simulink library "lib_TorqueDistribution_2017a"  (R2017a)
settings: Solver=VariableStepAuto  StartTime=0.0  StopTime=10.0  RelTol=1e-3
undefined symbols (not defined in the file): cal, eng, Engine, gb, mot
libraries: simulink x30, dspsigops x3, EC2_libraries x2
(part 1 of 4)
settings Model: Creator=Vraj M  LastModifiedBy=vraj

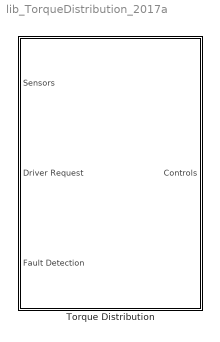
== system lib_TorqueDistribution_2017a ==
  Torque Distribution : Subsystem

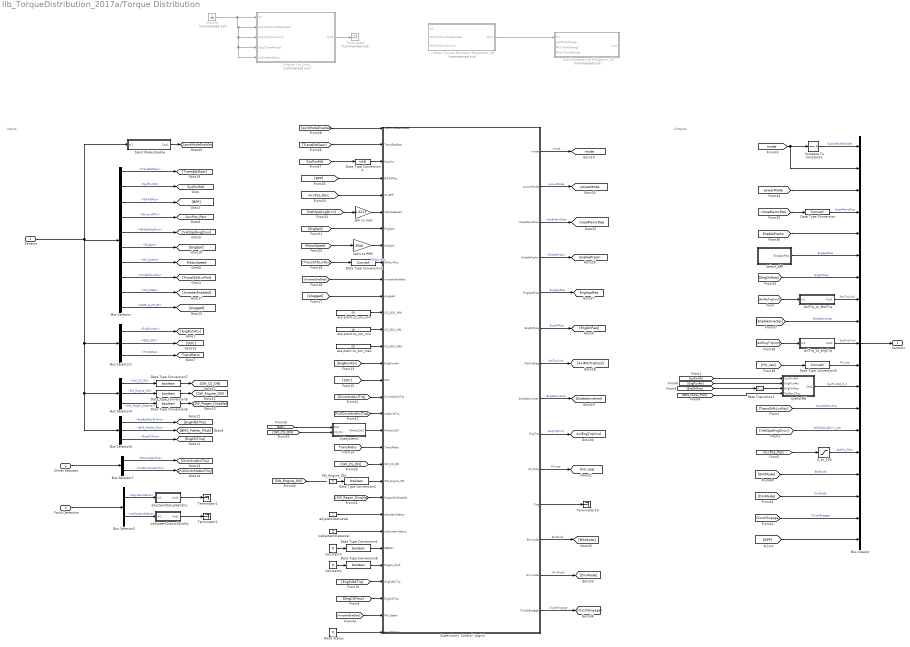
== system lib_TorqueDistribution_2017a/Torque Distribution ==
  note: Inputs
  note: Outputs
  Sensors : Inport
  Driver Request : Inport  Port=2
  Fault Detection : Inport  Port=3
  0_to_100 : Saturate  UpperLimit=100  LowerLimit=0
  AxlTrq_to_EngTrq : Subsystem
  AxlTrq_to_MotTrq : Subsystem
  Bus Creator : BusCreator  Inputs=19
  Bus Selector : BusSelector  OutputSignals=from_CAN.fromVEH_CAN.from_TCM.TransEstGear,from_CAN.fromVEH_CAN.from_BCM.SysPwrMd,from_CAN.fromVEH_CAN.from_BCM.BrkPdlPos,from_Analog.Driver_APP1,from_CAN.fromEBCAN.from_ECM.VehSpdAvgDrvn,from_CAN.fromEBCAN.from_ECM.EngSpd,from_CAN.fromHV_CAN.from_MCU.INV_VCU_01.INV_Speed,from_CAN.fromVEH_CAN.from_TCM.TrnsShftLvrPos,from_CAN.fromHV_CAN.from_MCU.INV_VCU_01.INV_State,from_CAN.fromHV_CAN.from_OBC.NLG5_ST.NLG5_S_CP_DT
  Bus Selector1 : BusSelector  OutputSignals=from_CAN.fromEBCAN.from_ECM.EngRunAtv,from_CAN.fromHV_CAN.from_BMSHybrid.BMS_SOC,from_CAN.fromVEH_CAN.from_TCM.TrnGrRat
  Bus Selector2 : BusSelector  OutputSignals=eSystemDiagOut.eSystemStatus,iceSystemDiagOut.iceSystemStatus
  Bus Selector4 : BusSelector  OutputSignals=from_Digital.SW_CS_ON,from_Digital.SW_Engine_ON,from_Digital.SW_Regen_Disable
  Bus Selector6 : BusSelector  OutputSignals=from_CAN.fromEBCAN.from_ECM.EngActStdyStTorq,from_CAN.fromHV_CAN.from_BMSHybrid.BMS_HYB_02.BMS_Fehler_Pilot,from_CAN.fromEBCAN.from_ECM.EngCltTmp
  Bus Selector7 : BusSelector  OutputSignals=DrvIntndAxlTrq,FullDrvIntndAxlTrq
  Compare To Constant1 : simulink/Logic and Bit Operations/Compare To Constant  relop===  const=4  OutDataTypeStr=boolean
  Constant2 : Constant  Value=0
  Constant3 : Constant  Value=0
  Data Type Conversion : DataTypeConversion
  Data Type Conversion{1..2,5..8} (6 alike) : DataTypeConversion  OutDataTypeStr=boolean
  Data Type Conversion3 : DataTypeConversion
  Data Type Conversion4 : DataTypeConversion  OutDataTypeStr=int8
  Data Type Conversion9 : DataTypeConversion
  Engine Trq Limit : Subsystem  Commented=on
  Ground : Ground  Commented=on
  Hood Status : Constant  Value=0
  Motor Troque Mismatch Mitigation_CD : Subsystem  Commented=on
  OverTemperature Mitigation_CD : Subsystem  Commented=on
  Rate Transition3 : RateTransition
  SW_Engine_ON : Constant  Value=0
  Select_APP : Subsystem
  Sport Mode Enable : Subsystem
  Subsystem1 : Subsystem
  Supervisory  Control  Logic1 : Stateflow chart  TreatAsAtomicUnit=on
  SysPwrMd : Subsystem
  Terminator : Terminator  Commented=on
  Terminator1 : Terminator
  Terminator10 : Terminator
  Terminator2 : Terminator
  eSystemStatusVal : Constant  Value=2
  eSystemStatusValidity : Subsystem
  ess.plant.cd_soc_min : Constant  Value=50
  ess.plant.cs_soc_max : Constant  Value=23
  ess.plant.cs_soc_min : Constant  Value=18
  iceSystemStatusVal : Constant  Value=2
  iceSystemStatusValidity : Subsystem
  kph to mph : Gain  Gain=0.6213
  rad/s to RPM : Gain  Gain=30/pi
  Controls : Outport
  tag scope: AccPos_Perc=global, AxlEngTrqCmd=global, EnablePrplsn=global, EngAppReq=global, MotorSpeed=global, SportModeEnabled=global, SysPwrMd=global, TransRatio=global, closeMaincReq=global, mode=global, powerMode=global
  wires:
  Hood Status/1 -> Supervisory  Control  Logic1/31(HoodStatus)
  Ground/1 -> Engine Trq Limit/1(In1), Engine Trq Limit/2(EngTrqMismchDegraded), Engine Trq Limit/3(EngTrqMismchLimp), Engine Trq Limit/4(Eng_TempRange), Engine Trq Limit/5(iceSystemStatus)
  [plugged] -> Supervisory  Control  Logic1/11(plugged)
  AxlTrq_to_EngTrq/1(Out1) -> Bus Creator/10  "EngTrqCmd"
  [closeMaincReq] -> Data Type Conversion/1
  Compare To Constant1/1 -> Bus Creator/1  "SportsModeEnable"
  [EngRunAtv] -> SysPwrMd/2(EngRunAtv)
  [ClutchEngage] -> Bus Creator/18  "ClutchEngage"
  [BPP] -> Bus Creator/19
  [AxlMtrTrqCmd] -> AxlTrq_to_MotTrq/1(In1)
  [AxlEngTrqCmd] -> AxlTrq_to_EngTrq/1(In1)
  [mode] -> Compare To Constant1/1, Bus Creator/2
  [TransShftLvrPos] -> Bus Creator/13  "TransShftLvrPos"
  [DrvMode] -> Bus Creator/17  "DrvMode"
  [SysPwrMd] -> SysPwrMd/1(SysPwrMd)
  SysPwrMd/1(Out1) -> Bus Creator/12  "SysPwrMd_0_3"
  [VehSpdAvgDrvn] -> Bus Creator/14  "VehSpdAvgDrvn_kph"
  Data Type Conversion9/1 -> Bus Creator/11  "HV_req"
  [BMS_Fehler_Pilot] -> SysPwrMd/4(Fehler_Pilot)
  [EnablePrplsn] -> Bus Creator/5
  [AccPos_Perc] -> 0_to_100/1
  [EnableInverter] -> Bus Creator/9  "EnableInverter"
  [EngOnReq] -> Bus Creator/7  "EngOnReq"
  [HV_req] -> Data Type Conversion9/1
  Select_APP/1(EngAppReq) -> Bus Creator/6  "EngAppReq"
  [BrkMode] -> Bus Creator/16  "BrkMode"
  AxlTrq_to_MotTrq/1(Out1) -> Bus Creator/8  "MtrTrqCmd"
  0_to_100/1 -> Bus Creator/15  "AccPos_Perc"
  [powerMode] -> Bus Creator/3
  Data Type Conversion/1 -> Bus Creator/4  "closeMaincReq"
  [EngOnReq] -> Rate Transition3/1
  Rate Transition3/1 -> SysPwrMd/3(EngOnReq)
  Bus Creator/1 -> Controls/1
  Sensors/1 -> Bus Selector/1, Sport Mode Enable/1(In1), Bus Selector1/1, Bus Selector4/1, Bus Selector6/1
  Bus Selector/1 -> [TransEstGear]  "<TransEstGear>"
  Bus Selector/2 -> [SysPwrMd]  "<SysPwrMd>"
  Bus Selector/3 -> [BPP]  "<BrkPdlPos>"
  Bus Selector/4 -> [AccPos_Perc]  "<Driver_APP1>"
  Bus Selector/5 -> [VehSpdAvgDrvn]  "<VehSpdAvgDrvn>"
  Bus Selector/6 -> [EngSpd]  "<EngSpd>"
  Bus Selector/7 -> [MotorSpeed]  "<INV_Speed>"
  Bus Selector/9 -> [InverterEnabled]  "<INV_State>"
  Bus Selector1/1 -> [EngRunAtv]  "<EngRunAtv>"
  Bus Selector/8 -> [TransShftLvrPos]  "<TrnsShftLvrPos>"
  Bus Selector1/3 -> [TransRatio]  "<TrnGrRat>"
  Fault Detection/1 -> Bus Selector2/1
  Bus Selector2/1 -> eSystemStatusValidity/1(In1)  "<eSystemStatus>"
  Bus Selector2/2 -> iceSystemStatusValidity/1(In1)  "<iceSystemStatus>"
  Bus Selector4/3 -> Data Type Conversion6/1  "<SW_Regen_Disable>"
  Bus Selector4/1 -> Data Type Conversion7/1  "<SW_CS_ON>"
  Bus Selector4/2 -> Data Type Conversion5/1  "<SW_Engine_ON>"
  eSystemStatusValidity/1(Out1) -> Terminator1/1
  iceSystemStatusValidity/1(Out1) -> Terminator2/1
  Bus Selector/10 -> [plugged]  "<NLG5_S_CP_DT>"
  Data Type Conversion5/1 -> [SW_Engine_ON]
  Data Type Conversion6/1 -> [SW_Regen_Disable]
  Bus Selector6/1 -> [EngFdbkTrq]  "<EngActStdyStTorq>"
  Bus Selector6/2 -> [BMS_Fehler_Pilot]  "<BMS_Fehler_Pilot>"
  Bus Selector6/3 -> [EngCltTmp]  "<EngCltTmp>"
  Bus Selector7/2 -> [FullDrvIntndAxlTrq]  "<FullDrvIntndAxlTrq>"
  Sport Mode Enable/1(Out1) -> [SportModeEnabled]
  Bus Selector1/2 -> [SOC]  "<BMS_SOC>"
  Data Type Conversion7/1 -> [SW_CS_ON]
  Driver Request/1 -> Bus Selector7/1
  Bus Selector7/1 -> [DrvIntndAxlTrq]  "<DrvIntndAxlTrq>"
  Supervisory  Control  Logic1/14(ClutchEngage) -> [ClutchEngage]  "ClutchEngage"
  Supervisory  Control  Logic1/13(Drvmode) -> [DrvMode]  "DrvMode"
  Supervisory  Control  Logic1/10(HV_Req) -> [HV_req]  "HV_req"
  Supervisory  Control  Logic1/9(EngTrq) -> [AxlEngTrqCmd]  "EngTrqCmd"
  Supervisory  Control  Logic1/7(MotTrqReq) -> [AxlMtrTrqCmd]  "MtrTrqCmd"
  Supervisory  Control  Logic1/6(EngOnReq) -> [EngOnReq]  "EngOnReq"
  [SW_CS_ON] -> Subsystem1/2(CS_On)
  [SW_Regen_Disable] -> Supervisory  Control  Logic1/23(RegenBrkDisable)
  [SW_Engine_ON] -> ?
  [SW_CS_ON] -> Supervisory  Control  Logic1/21(SW_CS_ON)
  [SportModeEnabled] -> Supervisory  Control  Logic1/1(SportModeEnabled)
  Data Type Conversion4/1 -> Supervisory  Control  Logic1/3(KeyPos)
  [SysPwrMd] -> Data Type Conversion4/1
  [TransEstGear] -> Supervisory  Control  Logic1/2(TransEstGear)
  [BPP] -> Supervisory  Control  Logic1/4(BrkPdlPos)
  [AccPos_Perc] -> Supervisory  Control  Logic1/5(drvAPP)
  [VehSpdAvgDrvn] -> kph to mph/1
  [EngSpd] -> Supervisory  Control  Logic1/7(EngSpd)
  [MotorSpeed] -> rad/s to RPM/1
  [TransShftLvrPos] -> Data Type Conversion3/1
  [InverterEnabled] -> Supervisory  Control  Logic1/10(InverterEnabled)
  [SOC] -> Subsystem1/1(SoC)
  [SOC] -> Supervisory  Control  Logic1/16(SoC)
  [TransRatio] -> Supervisory  Control  Logic1/20(TransRatio)
  [EngRunAtv] -> Supervisory  Control  Logic1/15(EngRunAtv)
  [EngFdbkTrq] -> Supervisory  Control  Logic1/28(EngFdbkTrq)
  [EngCltTmp] -> Supervisory  Control  Logic1/29(EngCtlTmp)
  rad/s to RPM/1 -> Supervisory  Control  Logic1/8(MotSpd)
  Supervisory  Control  Logic1/5(EngAppReq) -> [EngAppReq]  "EngAppReq"
  eSystemStatusVal/1 -> Supervisory  Control  Logic1/24(eSystemStatus)
  iceSystemStatusVal/1 -> Supervisory  Control  Logic1/25(iceSystemStatus)
  Data Type Conversion8/1 -> Supervisory  Control  Logic1/27(Regen_fault)
  Supervisory  Control  Logic1/12(Brkmode) -> [BrkMode]  "BrkMode"
  Subsystem1/1(Faked_SoC) -> Supervisory  Control  Logic1/19(Faked_SoC)
  Data Type Conversion1/1 -> Supervisory  Control  Logic1/26(ABSAtv)
  Constant3/1 -> Data Type Conversion1/1
  [FullDrvIntndAxlTrq] -> Supervisory  Control  Logic1/18(IntdAxleTrq)
  [DrvIntndAxlTrq] -> Supervisory  Control  Logic1/17(DrvIntdAxleTrq)
  Supervisory  Control  Logic1/11(Chg) -> Terminator10/1
  Motor Troque Mismatch Mitigation_CD/1(Out1) -> OverTemperature Mitigation_CD/1(In1)
  Engine Trq Limit/1(Out1) -> Terminator/1
  Constant2/1 -> Data Type Conversion8/1
  kph to mph/1 -> Supervisory  Control  Logic1/6(VehicleSpeed)
  Data Type Conversion3/1 -> Supervisory  Control  Logic1/9(ShftLvrPos)  "ShftLvrPos"
  Supervisory  Control  Logic1/1(mode) -> [mode]  "mode"
  Supervisory  Control  Logic1/2(powerMode) -> [powerMode]  "powerMode"
  Supervisory  Control  Logic1/3(closeMaincReq) -> [closeMaincReq]  "closeMaincReq"
  Supervisory  Control  Logic1/4(EnablePrplsn) -> [EnablePrplsn]  "EnablePrplsn"
  Supervisory  Control  Logic1/8(EnableInverter) -> [EnableInverter]  "EnableInverter"
  ess.plant.cs_soc_max/1 -> Supervisory  Control  Logic1/14(CS_SOC_MAX)
  ess.plant.cs_soc_min/1 -> Supervisory  Control  Logic1/13(CS_SOC_MIN)
  ess.plant.cd_soc_min/1 -> Supervisory  Control  Logic1/12(CD_SOC_MIN)
  SW_Engine_ON/1 -> Data Type Conversion2/1
  Data Type Conversion2/1 -> Supervisory  Control  Logic1/22(SW_Engine_ON)
  [InverterEnabled] -> Supervisory  Control  Logic1/30(INV_State)

== system lib_TorqueDistribution_2017a/Torque Distribution/AxlTrq_to_EngTrq ==
  note: //From engine axle torque to engine torque//
  note: check this rate limiter
  In1 : Inport
  Compare To Constant : simulink/Logic and Bit Operations/Compare To Constant  relop===  const=0  OutDataTypeStr=boolean
  Constant1 : Constant  Value=max(gb.plant.init.ratio.map)
  Constant5 : Constant  Value=fd.plant.init.ratio
  Divide1 : Product  Inputs=*//
  Ground : Ground  Commented=on
  Rate Limiter : RateLimiter  RisingSlewLimit=1000  FallingSlewLimit=-2000
  Rate Limiter1 : RateLimiter  Commented=on  RisingSlewLimit=Engine.trq_uprate  FallingSlewLimit=Engine.trq_derate
  Ratio Filter : Subsystem
  Switch : Switch  Criteria=u2 > Threshold
  Terminator : Terminator  Commented=on
  Out1 : Outport
  wires:
  Ground/1 -> Rate Limiter1/1
  Rate Limiter1/1 -> Terminator/1
  Ratio Filter/1(Filtered_Ratio) -> Compare To Constant/1, Switch/3
  Rate Limiter/1 -> Out1/1
  Switch/1 -> Divide1/3
  Constant1/1 -> Switch/1
  Compare To Constant/1 -> Switch/2
  [TransRatio] -> Ratio Filter/1(Ratio)
  Divide1/1 -> Rate Limiter/1
  Constant5/1 -> Divide1/2
  In1/1 -> Divide1/1

== system lib_TorqueDistribution_2017a/Torque Distribution/AxlTrq_to_MotTrq ==
  In1 : Inport
  AxlTrq_to_MtrTrq2 : Subsystem
  MotTrqLimit : Saturate  UpperLimit=250  LowerLimit=-200
  Scope : Scope  NumInputPorts=4
  Subsystem : Subsystem
  electric machine filter : Subsystem
  Out1 : Outport
  wires:
  [MotorSpeed] -> Subsystem/2(RPM)
  MotTrqLimit/1 -> Subsystem/1(In1), Scope/3  "MtrTrqCmd"
  Subsystem/1(Out1) -> Out1/1, Scope/4  "MtrTrqCmd"
  electric machine filter/1(filtered) -> MotTrqLimit/1, Scope/2  "MtrTrqCmd"
  AxlTrq_to_MtrTrq2/1(MtrTrqCmd) -> electric machine filter/1(trq), Scope/1  "MtrTrqCmd"
  In1/1 -> AxlTrq_to_MtrTrq2/1(In1)

== system lib_TorqueDistribution_2017a/Torque Distribution/Engine Trq Limit ==
  In1 : Inport
  EngTrqMismchDegraded : Inport  Port=2
  EngTrqMismchLimp : Inport  Port=3
  Eng_TempRange : Inport  Port=4
  iceSystemStatus : Inport  Port=5
  Compare To Constant : simulink/Logic and Bit Operations/Compare To Constant  relop===  const=1  OutDataTypeStr=boolean
  Eng Troque Mismatch Mitigation : Subsystem
  OverTemperature Mitigation : Subsystem
  Switch2 : Switch  Threshold=1
  Out1 : Outport
  wires:
  OverTemperature Mitigation/1(Out1) -> Switch2/1
  iceSystemStatus/1 -> Compare To Constant/1
  In1/1 -> Switch2/3, Eng Troque Mismatch Mitigation/1(In1)
  Eng Troque Mismatch Mitigation/1(Out1) -> OverTemperature Mitigation/1(In1)
  Eng_TempRange/1 -> OverTemperature Mitigation/2(essTempRange)
  EngTrqMismchDegraded/1 -> Eng Troque Mismatch Mitigation/2(EngTrqMismchDegraded)
  EngTrqMismchLimp/1 -> Eng Troque Mismatch Mitigation/3(EngTrqMismchLimp)
  Compare To Constant/1 -> Switch2/2
  Switch2/1 -> Out1/1

== system lib_TorqueDistribution_2017a/Torque Distribution/Motor Troque Mismatch Mitigation_CD ==
  In1 : Inport
  MotTrqMismchDegraded : Inport  Port=2
  MotTrqMismchLimp : Inport  Port=3
  Subsystem : Subsystem
  Out1 : Outport
  tag scope: TorqueRequest_Nm=global
  wires:
  Subsystem/1(Out1) -> Out1/1
  MotTrqMismchDegraded/1 -> Subsystem/2(In2)
  MotTrqMismchLimp/1 -> Subsystem/1(In1)
  In1/1 -> [TorqueRequest_Nm]

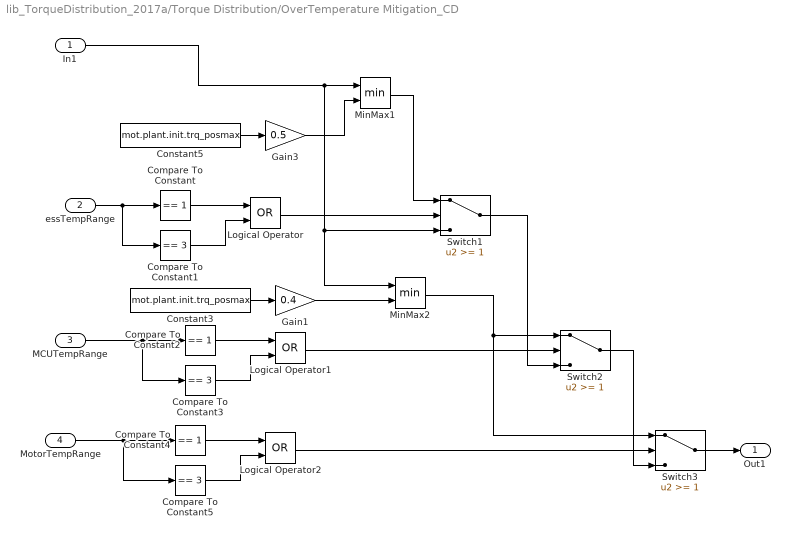
== system lib_TorqueDistribution_2017a/Torque Distribution/OverTemperature Mitigation_CD ==
  In1 : Inport
  essTempRange : Inport  Port=2
  MCUTempRange : Inport  Port=3
  MotorTempRange : Inport  Port=4
  Compare To Constant : simulink/Logic and Bit Operations/Compare To Constant  relop===  const=1  OutDataTypeStr=boolean
  Compare To Constant1 : simulink/Logic and Bit Operations/Compare To Constant  relop===  const=3  OutDataTypeStr=boolean
  Compare To Constant2 : simulink/Logic and Bit Operations/Compare To Constant  relop===  const=1  OutDataTypeStr=boolean
  Compare To Constant3 : simulink/Logic and Bit Operations/Compare To Constant  relop===  const=3  OutDataTypeStr=boolean
  Compare To Constant4 : simulink/Logic and Bit Operations/Compare To Constant  relop===  const=1  OutDataTypeStr=boolean
  Compare To Constant5 : simulink/Logic and Bit Operations/Compare To Constant  relop===  const=3  OutDataTypeStr=boolean
  Constant3 : Constant  Value=mot.plant.init.trq_posmax
  Constant5 : Constant  Value=mot.plant.init.trq_posmax
  Gain1 : Gain  Gain=0.4
  Gain3 : Gain  Gain=0.5
  Logical Operator : Logic  Operator=OR  AllPortsSameDT=off  OutDataTypeStr=boolean
  Logical Operator1 : Logic  Operator=OR  AllPortsSameDT=off  OutDataTypeStr=boolean
  Logical Operator2 : Logic  Operator=OR  AllPortsSameDT=off  OutDataTypeStr=boolean
  MinMax1 : MinMax  Inputs=2
  MinMax2 : MinMax  Inputs=2
  Switch1 : Switch  Threshold=1
  Switch2 : Switch  Threshold=1
  Switch3 : Switch  Threshold=1
  Out1 : Outport
  wires:
  Switch3/1 -> Out1/1
  Compare To Constant5/1 -> Logical Operator2/2
  Compare To Constant4/1 -> Logical Operator2/1
  Switch1/1 -> Switch2/3
  essTempRange/1 -> Compare To Constant/1, Compare To Constant1/1
  Compare To Constant3/1 -> Logical Operator1/2
  Compare To Constant2/1 -> Logical Operator1/1
  MCUTempRange/1 -> Compare To Constant2/1, Compare To Constant3/1
  Switch2/1 -> Switch3/3
  Gain3/1 -> MinMax1/2
  Gain1/1 -> MinMax2/2
  In1/1 -> MinMax1/1, Switch1/3, MinMax2/1
  Logical Operator2/1 -> Switch3/2
  Logical Operator/1 -> Switch1/2
  MinMax1/1 -> Switch1/1
  MinMax2/1 -> Switch2/1, Switch3/1
  Constant3/1 -> Gain1/1
  Compare To Constant/1 -> Logical Operator/1
  Compare To Constant1/1 -> Logical Operator/2
  Logical Operator1/1 -> Switch2/2
  Constant5/1 -> Gain3/1
  MotorTempRange/1 -> Compare To Constant4/1, Compare To Constant5/1

== system lib_TorqueDistribution_2017a/Torque Distribution/Select_APP ==
  APP_Select : Constant  Value=0
  Data Type Conversion10 : DataTypeConversion  OutDataTypeStr=boolean
  Switch1 : Switch  Criteria=u2 > Threshold
  EngAppReq : Outport
  wires:
  [EngAppReq] -> Switch1/3
  [AccPos_Perc] -> Switch1/1
  Data Type Conversion10/1 -> Switch1/2
  APP_Select/1 -> Data Type Conversion10/1
  Switch1/1 -> EngAppReq/1  "EngAppReq"

== system lib_TorqueDistribution_2017a/Torque Distribution/Sport Mode Enable ==
  In1 : Inport
  Bus Selector5 : BusSelector  OutputSignals=from_Analog.Sport_Mode_SW
  Compare To Constant : simulink/Logic and Bit Operations/Compare To Constant  relop===  const=2  OutDataTypeStr=boolean
  Sports Mode Logic : Stateflow chart  TreatAsAtomicUnit=on
  Out1 : Outport
  wires:
  In1/1 -> Bus Selector5/1
  Bus Selector5/1 -> Sports Mode Logic/1(Voltage_Input)  "<Sport_Mode_SW>"
  Sports Mode Logic/1(Driver_Mode) -> Compare To Constant/1
  Compare To Constant/1 -> Out1/1

== system lib_TorqueDistribution_2017a/Torque Distribution/Subsystem1 ==
  SoC : Inport
  CS_On : Inport  Port=2
  Constant : Constant
  Sample and Hold1 : dspsigops/Sample and Hold  trig=Rising edge  initCond=0  latchinput=off
  Switch : Switch  Criteria=u2 > Threshold
  Faked_SoC : Outport
  wires:
  SoC/1 -> Sample and Hold1/1
  CS_On/1 -> Switch/2, Sample and Hold1/Trigger
  Switch/1 -> Faked_SoC/1
  Sample and Hold1/1 -> Switch/1
  Constant/1 -> Switch/3

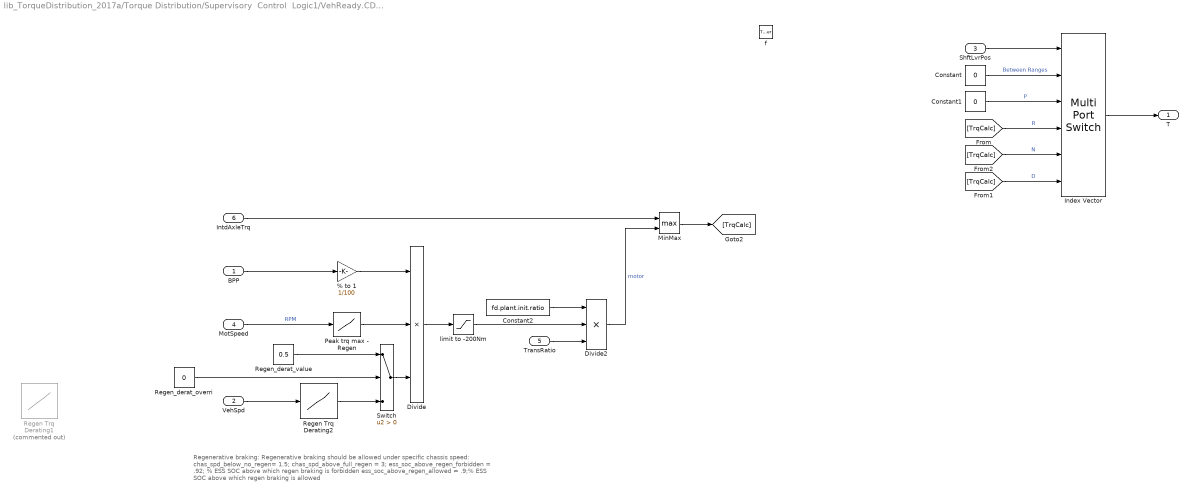
== system lib_TorqueDistribution_2017a/Torque Distribution/Supervisory  Control  Logic1/VehReady.CD_Mode.Brake_mode.MotTrqCalc1 ==
  note: Regenerative braking:
      | Regenerative braking should be allowed under specific chassis speed:
      | chas_spd_below_no_regen= 1.5;
      | chas_spd_above_full_regen = 3;
      | ess_soc_above_regen_forbidden = .92;  % ESS SOC above which regen braking is forbidden
      | ess_soc_above_regen_allowed = .9;% ESS SOC above which regen braking is allowed
  BPP : Inport
  VehSpd : Inport  Port=2
  ShftLvrPos : Inport  Port=3
  MotSpeed : Inport  Port=4
  TransRatio : Inport  Port=5
  IntdAxleTrq : Inport  Port=6
  f : TriggerPort  TriggerType=function-call  VariantControl=Variant
      settings: CopyFcn=Stateflow.SLINSF.SimulinkMan.removeBlockPreDeleteFcn  PreDeleteFcn=Stateflow.SLINSF.SimulinkMan.unsafePredeleteFcn
  "% to 1 " : Gain  Gain=1/100
  Constant : Constant  Value=0
  Constant1 : Constant  Value=0
  Constant2 : Constant  Value=fd.plant.init.ratio
  Divide : Product  Inputs=***
  Divide2 : Product  Inputs=***
  Index Vector : MultiPortSwitch  DataPortOrder=Zero-based contiguous  Inputs=5  zeroidx=on
  MinMax : MinMax  Function=max  Inputs=2
  Peak trq max - Regen : Lookup  InputValues=mot.plant.init.regen.trq_max.idx1_spd  Table=mot.plant.init.regen.trq_max.map  LookUpMeth=Interpolation-Use End Values  SaturateOnIntegerOverflow=on
  Regen Trq Derating1 : Lookup_n-D  Commented=on  NumberOfTableDimensions=1  BreakpointsForDimension1=[0 10 20 30 40]  Table=[0 0.025 0.05 0.1 1]  ExtrapMethod=Clip  UseLastTableValue=on  InternalRulePriority=Speed  RndMeth=Simplest  InputSameDT=on
  Regen Trq Derating2 : Lookup_n-D  NumberOfTableDimensions=1  BreakpointsForDimension1=[0 10 11 200]  Table=[0 0.5 1 1]  ExtrapMethod=Clip  UseLastTableValue=on  InternalRulePriority=Speed  RndMeth=Simplest  InputSameDT=on
  Regen_derat_overri : Constant  Value=0
  Regen_derat_value : Constant  Value=0.5
  Switch : Switch  Criteria=u2 > Threshold
  limit to -200Nm : Saturate  UpperLimit=0  LowerLimit=-200
  T : Outport
  wires:
  MinMax/1 -> [TrqCalc]
  IntdAxleTrq/1 -> MinMax/1
  Regen_derat_value/1 -> Switch/1
  Switch/1 -> Divide/3
  Regen_derat_overri/1 -> Switch/2
  Regen Trq Derating2/1 -> Switch/3
  Divide2/1 -> MinMax/2  "motor"
  TransRatio/1 -> Divide2/3
  limit to -200Nm/1 -> Divide2/2
  Constant2/1 -> Divide2/1
  Peak trq max - Regen/1 -> Divide/2
  MotSpeed/1 -> Peak trq max - Regen/1  "RPM"
  [TrqCalc] -> Index Vector/5  "N"
  Constant1/1 -> Index Vector/3  "P"
  Constant/1 -> Index Vector/2  "Between Ranges"
  Index Vector/1 -> T/1
  [TrqCalc] -> Index Vector/6  "D"
  [TrqCalc] -> Index Vector/4  "R"
  ShftLvrPos/1 -> Index Vector/1
  VehSpd/1 -> Regen Trq Derating2/1
  Divide/1 -> limit to -200Nm/1
  "% to 1 "/1 -> Divide/1
  BPP/1 -> "% to 1 "/1

== system lib_TorqueDistribution_2017a/Torque Distribution/Supervisory  Control  Logic1/VehReady.CD_Mode.Brake_mode.MotTrqCalc2 ==
  note: Regenerative braking:
      | Regenerative braking should be allowed under specific chassis speed:
      | chas_spd_below_no_regen= 1.5;
      | chas_spd_above_full_regen = 3;
      | ess_soc_above_regen_forbidden = .92;  % ESS SOC above which regen braking is forbidden
      | ess_soc_above_regen_allowed = .9;% ESS SOC above which regen braking is allowed
  ShftLvrPos : Inport
  TransRatio : Inport  Port=2
  f : TriggerPort  TriggerType=function-call  VariantControl=Variant
      settings: CopyFcn=Stateflow.SLINSF.SimulinkMan.removeBlockPreDeleteFcn  PreDeleteFcn=Stateflow.SLINSF.SimulinkMan.unsafePredeleteFcn
  Constant : Constant  Value=0
  Constant1 : Constant  Value=0
  Constant2 : Constant  Value=fd.plant.init.ratio
  Divide2 : Product  Inputs=***
  Idle_torque_Regen : Constant  Value=0
  Index Vector : MultiPortSwitch  DataPortOrder=Zero-based contiguous  Inputs=5  zeroidx=on
  T : Outport
  wires:
  Idle_torque_Regen/1 -> Divide2/2
  Divide2/1 -> [TrqCalc]  "motor"
  TransRatio/1 -> Divide2/3
  Constant2/1 -> Divide2/1
  [TrqCalc] -> Index Vector/5  "N"
  Constant1/1 -> Index Vector/3  "P"
  Constant/1 -> Index Vector/2  "Between Ranges"
  Index Vector/1 -> T/1
  [TrqCalc] -> Index Vector/6  "D"
  [TrqCalc] -> Index Vector/4  "R"
  ShftLvrPos/1 -> Index Vector/1

== system lib_TorqueDistribution_2017a/Torque Distribution/Supervisory  Control  Logic1/VehReady.CD_Mode.Drive_mode.MotTrqCalc2 ==
  APP : Inport
  ShftLvrPos : Inport  Port=2
  DrvIntdAxleTrq : Inport  Port=3
  TransRatio : Inport  Port=4
  f : TriggerPort  TriggerType=function-call  VariantControl=Variant
      settings: CopyFcn=Stateflow.SLINSF.SimulinkMan.removeBlockPreDeleteFcn  PreDeleteFcn=Stateflow.SLINSF.SimulinkMan.unsafePredeleteFcn
  Constant : Constant  Value=0
  Constant1 : Constant  Value=0
  Constant2 : Constant  Value=0
  Constant4 : Constant  Value=fd.plant.init.ratio
  Divide2 : Product  Inputs=***
  Index Vector : MultiPortSwitch  DataPortOrder=Zero-based contiguous  Inputs=5  zeroidx=on
  MinMax : MinMax  Inputs=2
  No Torque : Constant  Value=0
  Switch : Switch  Criteria=u2 > Threshold
  drvAPP2CmbTrq : Lookup_n-D  NumberOfTableDimensions=1  BreakpointsForDimension1=[0:1:100]  Table="[5.56903344175488\t20.4825939726242\t30.8750936087224\t37.8858960156155\t42.4930407106164\t45.5262617447488\t47.6795267594729\t49.5230964181710\t51.5151042123953\t54.0126566428754\t57.2824537752881\t61.5109301707869\t66.8139161912932\t73.2458196795481\t80.8083280139256\t89.4586305380063\t99.1171613649123\t109.674862556403\t120.999967676731\t132.944305721263\t145.349125419852\t158.050439914986\t170.883891814679\t183.689138620140\t196.313758528191\t208.616676608453\t220.471111355289\t231.767041614511\t242.413193884843\t252.338549994152\t261.493375150436\t269.849766367567\t277.401721265812\t284.164727247094\t290.174871045030\t295.487468649722\t300.175215607313\t304.325857694294\t308.039381966595\t311.424728183407\t314.596020605783\t317.668320170009\t320.752897035709\t323.952023508727\t327.353287338782\t331.023425391852\t335.001677697353\t339.292661870046\t343.858767906758\t348.612073357775\t353.405778873103\t358.025164123398\t362.178064095715\t365.484865763984\t367.468025134290\t367.541104664833\t364.997331060762\t364.997331060762\t364.997331060762\t364.997331060762\t364.997331060762\t364.997331060762\t364.997331060762\t364.997331060762\t364.997331060762\t364.997331060762\t364.997331060762\t364.997331060762\t364.997331060762\t364.997331060762\t364.997331060762\t364.997331060762\t364.997331060762\t364.997331060762\t364.997331060762\t364.997331060762\t364.997331060762\t364.997331060762\t364.997331060762\t364.997331060762\t364.997331060762\t364.997331060762\t364.997331060762\t364.997331060762\t364.997331060762\t364.997331060762\t364.997331060762\t364.997331060762\t364.997331060762\t364.997331060762\t364.997331060762\t364.997331060762\t364.997331060762\t364.997331060762\t364.997331060762\t364.997331060762\t364.997331060762\t364.997331060762\t364.997331060762\t364.997331060762\t364.997331060762]"  ExtrapMethod=Clip  UseLastTableValue=on  InternalRulePriority=Speed  RndMeth=Simplest  InputSameDT=on
  MotTrq : Outport
  wires:
  drvAPP2CmbTrq/1 -> Divide2/3
  MinMax/1 -> [TrqCalc]
  No Torque/1 -> Switch/3
  TransRatio/1 -> Divide2/1
  Switch/1 -> MinMax/2  "MotAvlTrq"
  Divide2/1 -> Switch/1
  DrvIntdAxleTrq/1 -> MinMax/1
  APP/1 -> drvAPP2CmbTrq/1, Switch/2
  Constant4/1 -> Divide2/2
  Index Vector/1 -> MotTrq/1
  Constant2/1 -> Index Vector/5  "N"
  Constant1/1 -> Index Vector/3  "P"
  Constant/1 -> Index Vector/2  "Between Ranges"
  [TrqCalc] -> Index Vector/6  "D"
  [TrqCalc] -> Index Vector/4  "R"
  ShftLvrPos/1 -> Index Vector/1

== system lib_TorqueDistribution_2017a/Torque Distribution/Supervisory  Control  Logic1/VehReady.CS_Mode.Clutch_Engage.SyncCtrl ==
  EngSpeed : Inport
  MotorSpeed : Inport  Port=2
  f : TriggerPort  TriggerType=function-call  VariantControl=Variant
      settings: CopyFcn=Stateflow.SLINSF.SimulinkMan.removeBlockPreDeleteFcn  PreDeleteFcn=Stateflow.SLINSF.SimulinkMan.unsafePredeleteFcn
  Kp : Gain  Gain=1/100
  Saturation : Saturate  UpperLimit=20  LowerLimit=0
  Scope : Scope  NumInputPorts=2
  Sum : Sum  Inputs=|+-
  EngApp : Outport
  wires:
  Saturation/1 -> EngApp/1
  Kp/1 -> Saturation/1
  Sum/1 -> Kp/1
  EngSpeed/1 -> Sum/2, Scope/2
  MotorSpeed/1 -> Sum/1, Scope/1  "RPM"

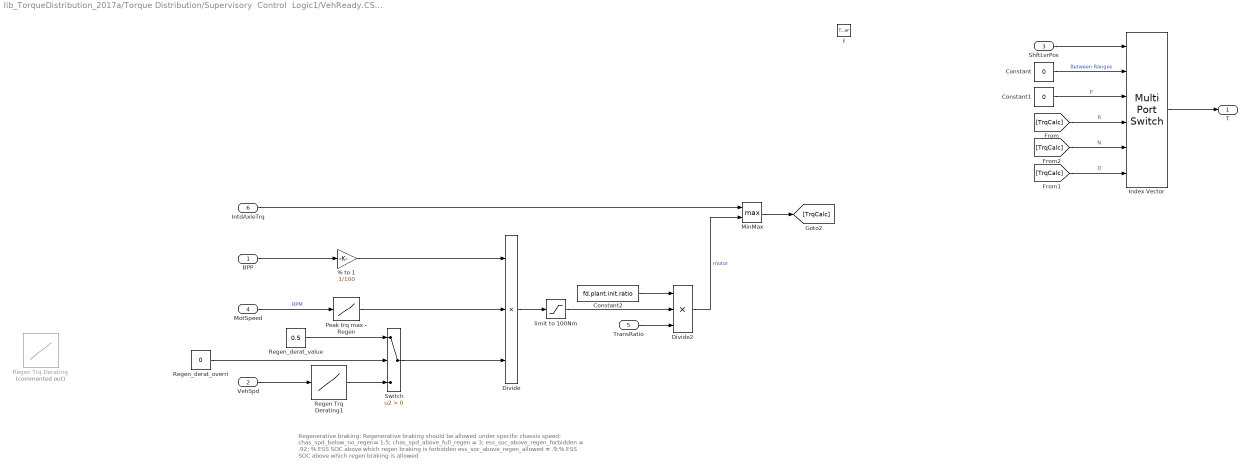
== system lib_TorqueDistribution_2017a/Torque Distribution/Supervisory  Control  Logic1/VehReady.CS_Mode.Engine_Charge.Brake_mode1.MotTrqCalc1 ==
  note: Regenerative braking:
      | Regenerative braking should be allowed under specific chassis speed:
      | chas_spd_below_no_regen= 1.5;
      | chas_spd_above_full_regen = 3;
      | ess_soc_above_regen_forbidden = .92;  % ESS SOC above which regen braking is forbidden
      | ess_soc_above_regen_allowed = .9;% ESS SOC above which regen braking is allowed
  BPP : Inport
  VehSpd : Inport  Port=2
  ShftLvrPos : Inport  Port=3
  MotSpeed : Inport  Port=4
  TransRatio : Inport  Port=5
  IntdAxleTrq : Inport  Port=6
  f : TriggerPort  TriggerType=function-call  VariantControl=Variant
      settings: CopyFcn=Stateflow.SLINSF.SimulinkMan.removeBlockPreDeleteFcn  PreDeleteFcn=Stateflow.SLINSF.SimulinkMan.unsafePredeleteFcn
  "% to 1 " : Gain  Gain=1/100
  Constant : Constant  Value=0
  Constant1 : Constant  Value=0
  Constant2 : Constant  Value=fd.plant.init.ratio
  Divide : Product  Inputs=***
  Divide2 : Product  Inputs=***
  Index Vector : MultiPortSwitch  DataPortOrder=Zero-based contiguous  Inputs=5  zeroidx=on
  MinMax : MinMax  Function=max  Inputs=2
  Peak trq max - Regen : Lookup  InputValues=mot.plant.init.regen.trq_max.idx1_spd  Table=mot.plant.init.regen.trq_max.map  LookUpMeth=Interpolation-Use End Values  SaturateOnIntegerOverflow=on
  Regen Trq Derating : Lookup_n-D  Commented=on  NumberOfTableDimensions=1  BreakpointsForDimension1=[0 20 30 40 50]  Table=[0 0.025 0.05 0.1 1]  ExtrapMethod=Clip  UseLastTableValue=on  InternalRulePriority=Speed  RndMeth=Simplest  InputSameDT=on
  Regen Trq Derating1 : Lookup_n-D  NumberOfTableDimensions=1  BreakpointsForDimension1=[0 10 11 200]  Table=[0 0.5 1 1]  ExtrapMethod=Clip  UseLastTableValue=on  InternalRulePriority=Speed  RndMeth=Simplest  InputSameDT=on
  Regen_derat_overri : Constant  Value=0
  Regen_derat_value : Constant  Value=0.5
  Switch : Switch  Criteria=u2 > Threshold
  limit to 100Nm : Saturate  UpperLimit=0  LowerLimit=-100
  T : Outport
  wires:
  MinMax/1 -> [TrqCalc]
  IntdAxleTrq/1 -> MinMax/1
  Regen_derat_value/1 -> Switch/1
  Switch/1 -> Divide/3
  Regen_derat_overri/1 -> Switch/2
  Regen Trq Derating1/1 -> Switch/3
  Divide2/1 -> MinMax/2  "motor"
  TransRatio/1 -> Divide2/3
  limit to 100Nm/1 -> Divide2/2
  Constant2/1 -> Divide2/1
  Peak trq max - Regen/1 -> Divide/2
  MotSpeed/1 -> Peak trq max - Regen/1  "RPM"
  [TrqCalc] -> Index Vector/5  "N"
  Constant1/1 -> Index Vector/3  "P"
  Constant/1 -> Index Vector/2  "Between Ranges"
  Index Vector/1 -> T/1
  [TrqCalc] -> Index Vector/6  "D"
  [TrqCalc] -> Index Vector/4  "R"
  ShftLvrPos/1 -> Index Vector/1
  VehSpd/1 -> Regen Trq Derating1/1
  Divide/1 -> limit to 100Nm/1
  "% to 1 "/1 -> Divide/1
  BPP/1 -> "% to 1 "/1

== system lib_TorqueDistribution_2017a/Torque Distribution/Supervisory  Control  Logic1/VehReady.CS_Mode.Engine_Charge.Brake_mode1.MotTrqCalc2 ==
  note: Regenerative braking:
      | Regenerative braking should be allowed under specific chassis speed:
      | chas_spd_below_no_regen= 1.5;
      | chas_spd_above_full_regen = 3;
      | ess_soc_above_regen_forbidden = .92;  % ESS SOC above which regen braking is forbidden
      | ess_soc_above_regen_allowed = .9;% ESS SOC above which regen braking is allowed
  ShftLvrPos : Inport
  TransRatio : Inport  Port=2
  f : TriggerPort  TriggerType=function-call  VariantControl=Variant
      settings: CopyFcn=Stateflow.SLINSF.SimulinkMan.removeBlockPreDeleteFcn  PreDeleteFcn=Stateflow.SLINSF.SimulinkMan.unsafePredeleteFcn
  Constant : Constant  Value=0
  Constant1 : Constant  Value=0
  Constant2 : Constant  Value=fd.plant.init.ratio
  Divide2 : Product  Inputs=***
  Idle_torque_Regen : Constant  Value=0
  Index Vector : MultiPortSwitch  DataPortOrder=Zero-based contiguous  Inputs=5  zeroidx=on
  T : Outport
  wires:
  Idle_torque_Regen/1 -> Divide2/2
  Divide2/1 -> [TrqCalc]  "motor"
  TransRatio/1 -> Divide2/3
  Constant2/1 -> Divide2/1
  [TrqCalc] -> Index Vector/5  "N"
  Constant1/1 -> Index Vector/3  "P"
  Constant/1 -> Index Vector/2  "Between Ranges"
  Index Vector/1 -> T/1
  [TrqCalc] -> Index Vector/6  "D"
  [TrqCalc] -> Index Vector/4  "R"
  ShftLvrPos/1 -> Index Vector/1

== system lib_TorqueDistribution_2017a/Torque Distribution/Supervisory  Control  Logic1/VehReady.CS_Mode.Engine_Charge.Drive_Mode.EngTrq2EngApp ==
  Trq : Inport
  TransRatio : Inport  Port=2
  f : TriggerPort  TriggerType=function-call  VariantControl=Variant
      settings: CopyFcn=Stateflow.SLINSF.SimulinkMan.removeBlockPreDeleteFcn  PreDeleteFcn=Stateflow.SLINSF.SimulinkMan.unsafePredeleteFcn
  APPCALCSWT : Constant
  Compare To Constant : simulink/Logic and Bit Operations/Compare To Constant  relop===  const=0  OutDataTypeStr=boolean
  Constant1 : Constant  Value=eps
  Constant2 : Constant  Value=231
  Constant5 : Constant  Value=fd.plant.init.ratio
  Divide : Product  Inputs=*/
  Divide1 : Product  Inputs=*//
  EngTrq2EngAPP : Lookup_n-D  NumberOfTableDimensions=1  BreakpointsForDimension1=[0:1:230]  Table="[-0.950562242591810\t-0.861179388327002\t-0.757792747831397\t-0.640901927898975\t-0.511000095283862\t-0.368573976700328\t-0.214103858822793\t-0.0480635882858183\t0.129079428315885\t0.316864224427463\t0.514836273533913\t0.722547489160089\t0.939556224870697\t1.16542727427030\t1.39973187100331\t1.64204768875400\t1.89195884124648\t2.14905588224475\t2.41293580555262\t2.68320204501379\t2.95946447451180\t3.24133940797003\t3.52844959935174\t3.82042424266002\t4.11689897193784\t4.41751586126800\t4.72192342477317\t5.02977661661586\t5.34073683099846\t5.65447190216317\t5.97065610439209\t6.28897015200715\t6.60910119937013\t6.93074284088268\t7.25359511098630\t7.57736448416234\t7.90176387493200\t8.22651263785634\t8.55133656753627\t8.87596789861257\t9.20014530576584\t9.52361390371657\t9.84612524722509\t10.1674373310916\t10.4873145901561\t10.8055278992985\t11.1218545734385\t11.4360783675358\t11.7479894765898\t12.0573845356398\t12.3640666197649\t12.6678452440843\t12.9685363637566\t13.2659623739808\t13.5599521099953\t13.8503408470787\t14.1369703005491\t14.4196886257647\t14.6983504181235\t14.9728167130634\t15.2429549860620\t15.5086391526369\t15.7697495683456\t16.0261730287853\t16.2778027695931\t16.5245384664460\t16.7662862350608\t17.0029586311942\t17.2344746506427\t17.4607597292427\t17.6817457428705\t17.8973710074422\t18.1075802789137\t18.3123247532808\t18.5115620665792\t18.7052562948843\t18.8933779543117\t19.0759040010164\t19.2528178311935\t19.4241092810781\t19.5897746269448\t19.7498165851084\t19.9042443119232\t20.0530734037837\t20.1963258971241\t20.3340302684184\t20.4662214341804\t20.5929407509641\t20.7142360153630\t20.8301614640105\t20.9407777735800\t21.0461520607847\t21.1463578823776\t21.2414752351516\t21.3315905559394\t21.4167967216136\t21.4971930490867\t21.5728852953111\t21.6439856572787\t21.7106127720217\t21.7728917166119\t21.8309540081611\t21.8849376038208\t21.9349869007824\t21.9812527362772\t22.0238923875764\t22.0630695719909\t22.0989544468717\t22.1317236096093\t22.1615600976344\t22.1886533884173\t22.2131993994684\t22.2354004883376\t22.2554654526151\t22.2736095299306\t22.2900543979538\t22.3050281743942\t22.3187654170013\t22.3315071235641\t22.3435007319120\t22.3550001199137\t22.3662656054781\t22.3775639465539\t22.3891683411296\t22.4013584272335\t22.4144202829338\t22.4286464263386\t22.4443358155959\t22.4617938488934\t22.4813323644587\t22.5032696405595\t22.5279303955028\t22.5556457876361\t22.5867534153463\t22.6215973170604\t22.6605279712450\t22.7039022964069\t22.7520836510924\t22.8054418338880\t22.8643530834197\t22.9292000783536\t23.0003719373956\t23.0782642192915\t23.1632789228268\t23.2558244868269\t23.3563157901571\t23.4651741517227\t23.5828273304686\t23.7097095253797\t23.8462613754808\t23.9929299598362\t24.1501687975506\t24.3184378477682\t24.4982035096730\t24.6899386224892\t24.8941224654804\t25.1112407579505\t25.3417856592430\t25.5862557687413\t25.8451561258686\t26.1189982100880\t26.4082999409026\t26.7135856778550\t27.0353862205281\t27.3742388085443\t27.7306871215661\t28.1052812792955\t28.4985778414748\t28.9111398078859\t29.3435366183506\t29.7963441527305\t30.2701447309271\t30.7655271128819\t31.2830864985759\t31.8234245280303\t32.3871492813060\t32.9748752785038\t33.5872234797643\t34.2248212852680\t34.8883025352352\t35.5783075099261\t36.2954829296408\t37.0404819547192\t37.8139641855409\t38.6165956625258\t39.4490488661331\t40.3120027168621\t41.2061425752523\t42.1321602418824\t43.0907539573713\t44.0826284023780\t45.1084946976008\t46.1690704037782\t47.2650795216887\t48.3972524921501\t49.5663261960208\t50.7730439541983\t52.0181555276205\t53.3024171172650\t54.6265913641491\t55.9914473493301\t57.3977605939052\t58.8463130590113\t60.3378931458253\t61.8732956955639\t63.4533219894835\t65.0787797488808\t66.7504831350916\t68.4692527494924\t70.2359156334991\t72.0513052685674\t73.9162615761929\t75.8316309179113\t77.7982660952979\t79.8170263499681\t81.8887773635766\t84.0143912578187\t86.1947465944290\t88.4307283751822\t90.7232280418928\t93.0731434764153\t95.4813790006436\t97.9488453765121\t100\t100\t100\t100\t100\t100\t100\t100]"  ExtrapMethod=Clip  UseLastTableValue=on  InternalRulePriority=Speed  RndMeth=Simplest  InputSameDT=on
  Gain : Gain  Gain=100
  Saturation : Saturate  UpperLimit=100  LowerLimit=0
  Switch : Switch  Criteria=u2 > Threshold
  Switch1 : Switch  Criteria=u2 > Threshold
  APP : Outport
  wires:
  Gain/1 -> Switch1/3
  APPCALCSWT/1 -> Switch1/2
  EngTrq2EngAPP/1 -> Switch1/1
  Divide/1 -> Gain/1
  Constant2/1 -> Divide/2
  Saturation/1 -> APP/1
  Switch1/1 -> Saturation/1
  TransRatio/1 -> Compare To Constant/1, Switch/3
  Divide1/1 -> EngTrq2EngAPP/1, Divide/1  "CSEngTrqCmd"
  Switch/1 -> Divide1/3
  Constant1/1 -> Switch/1
  Compare To Constant/1 -> Switch/2
  Constant5/1 -> Divide1/2
  Trq/1 -> Divide1/1  "CSEngAxlTrqCmd"

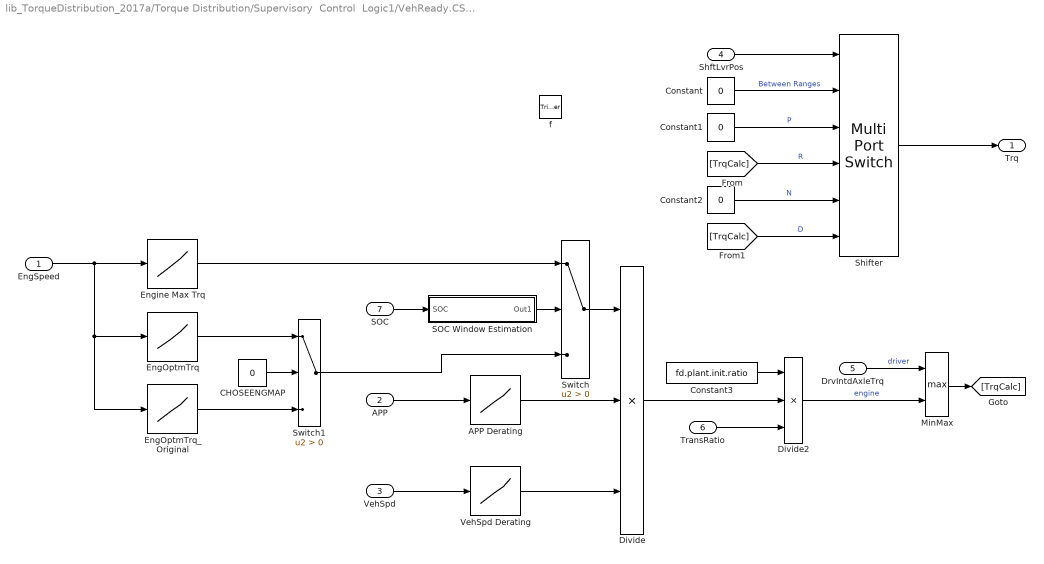
== system lib_TorqueDistribution_2017a/Torque Distribution/Supervisory  Control  Logic1/VehReady.CS_Mode.Engine_Charge.Drive_Mode.EngTrqCalc ==
  EngSpeed : Inport
  APP : Inport  Port=2
  VehSpd : Inport  Port=3
  ShftLvrPos : Inport  Port=4
  DrvIntdAxleTrq : Inport  Port=5
  TransRatio : Inport  Port=6
  SOC : Inport  Port=7
  f : TriggerPort  TriggerType=function-call  VariantControl=Variant
      settings: CopyFcn=Stateflow.SLINSF.SimulinkMan.removeBlockPreDeleteFcn  PreDeleteFcn=Stateflow.SLINSF.SimulinkMan.unsafePredeleteFcn
  APP Derating : Lookup_n-D  NumberOfTableDimensions=1  BreakpointsForDimension1=[0 1 2 3 5 7]  Table=[0 0.1 0.3 0.5 0.7 1]  ExtrapMethod=Clip  UseLastTableValue=on  InternalRulePriority=Speed  RndMeth=Simplest  InputSameDT=on
  CHOSEENGMAP : Constant  Value=0
  Constant : Constant  Value=0
  Constant1 : Constant  Value=0
  Constant2 : Constant  Value=0
  Constant3 : Constant  Value=fd.plant.init.ratio
  Divide : Product  Inputs=***
  Divide2 : Product  Inputs=***
  EngOptmTrq : Lookup_n-D  NumberOfTableDimensions=1  BreakpointsForDimension1=[850 1050 1300 1550 1650 1850 2050 2350 2650 2950 3150 3250 3350]  Table="[60 80 120 154.020912669576\t173.623574282068\t180.662367834043\t186.327738253926\t182.858870786433\t180.175407273844\t178.037732950256\t181.891363533595\t190.985931710274\t199.537540592824]"  ExtrapMethod=Clip  UseLastTableValue=on  InternalRulePriority=Speed  RndMeth=Simplest  InputSameDT=on
  EngOptmTrq_Original : Lookup_n-D  NumberOfTableDimensions=1  BreakpointsForDimension1=[1550 1650 1850 2050 2350 2650 2950 3150 3250 3350]  Table="[154.020912669576\t173.623574282068\t180.662367834043\t186.327738253926\t182.858870786433\t180.175407273844\t178.037732950256\t181.891363533595\t190.985931710274\t199.537540592824]"  ExtrapMethod=Clip  UseLastTableValue=on  InternalRulePriority=Speed  RndMeth=Simplest  InputSameDT=on
  Engine Max Trq : Lookup_n-D  NumberOfTableDimensions=1  BreakpointsForDimension1="[600\t800\t1000\t1200\t1400\t1600\t1800\t2000\t2200\t2400\t2600\t2800\t3000\t3200\t3400\t3600\t3800\t4000\t4250\t4500\t4750\t5000\t5250\t5500\t5750\t6000\t6250\t6500]"  Table="[83.7900000000000\t136.760000000000\t140\t152.010000000000\t171.590000000000\t185.900000000000\t198.400000000000\t197.360000000000\t200.550000000000\t202.260000000000\t215.080000000000\t204.810000000000\t204.520000000000\t208.100000000000\t211.520000000000\t210.560000000000\t214.100000000000\t213.470000000000\t208.730000000000\t208.430000000000\t208.670000000000\t231.210000000000\t228.310000000000\t225.330000000000\t220.520000000000\t211.210000000000\t204.190000000000\t151.770000000000]"  ExtrapMethod=Clip  UseLastTableValue=on  InternalRulePriority=Speed  RndMeth=Simplest  InputSameDT=on
  MinMax : MinMax  Function=max  Inputs=2
  SOC Window Estimation : Subsystem
  Shifter : MultiPortSwitch  DataPortOrder=Zero-based contiguous  Inputs=5  zeroidx=on
  Switch : Switch  Criteria=u2 > Threshold
  Switch1 : Switch  Criteria=u2 > Threshold
  VehSpd Derating : Lookup_n-D  NumberOfTableDimensions=1  BreakpointsForDimension1=[0 2 5]  Table=[0 0.5 1]  ExtrapMethod=Clip  UseLastTableValue=on  InternalRulePriority=Speed  RndMeth=Simplest  InputSameDT=on
  Trq : Outport
  wires:
  CHOSEENGMAP/1 -> Switch1/2
  EngOptmTrq_Original/1 -> Switch1/3
  Switch1/1 -> Switch/3
  EngOptmTrq/1 -> Switch1/1
  Engine Max Trq/1 -> Switch/1
  SOC Window Estimation/1(Out1) -> Switch/2
  SOC/1 -> SOC Window Estimation/1(SOC)
  Switch/1 -> Divide/1
  MinMax/1 -> [TrqCalc]
  DrvIntdAxleTrq/1 -> MinMax/1  "driver"
  TransRatio/1 -> Divide2/3
  Divide2/1 -> MinMax/2  "engine"
  Divide/1 -> Divide2/2
  Constant3/1 -> Divide2/1
  Shifter/1 -> Trq/1
  Constant2/1 -> Shifter/5  "N"
  Constant1/1 -> Shifter/3  "P"
  Constant/1 -> Shifter/2  "Between Ranges"
  [TrqCalc] -> Shifter/6  "D"
  [TrqCalc] -> Shifter/4  "R"
  ShftLvrPos/1 -> Shifter/1
  VehSpd Derating/1 -> Divide/3
  VehSpd/1 -> VehSpd Derating/1
  APP Derating/1 -> Divide/2
  APP/1 -> APP Derating/1
  EngSpeed/1 -> EngOptmTrq/1, EngOptmTrq_Original/1, Engine Max Trq/1

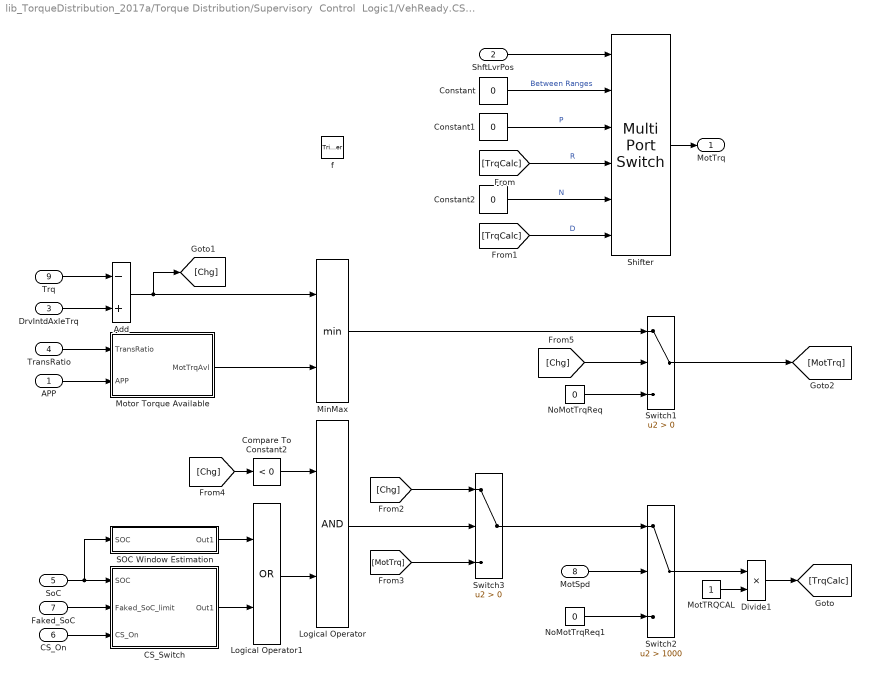
== system lib_TorqueDistribution_2017a/Torque Distribution/Supervisory  Control  Logic1/VehReady.CS_Mode.Engine_Charge.Drive_Mode.MotTrqCalc2 ==
  APP : Inport
  ShftLvrPos : Inport  Port=2
  DrvIntdAxleTrq : Inport  Port=3
  TransRatio : Inport  Port=4
  SoC : Inport  Port=5
  CS_On : Inport  Port=6
  Faked_SoC : Inport  Port=7
  MotSpd : Inport  Port=8
  Trq : Inport  Port=9
  f : TriggerPort  TriggerType=function-call  VariantControl=Variant
      settings: CopyFcn=Stateflow.SLINSF.SimulinkMan.removeBlockPreDeleteFcn  PreDeleteFcn=Stateflow.SLINSF.SimulinkMan.unsafePredeleteFcn
  Add : Sum  Inputs=-+
  CS_Switch : Subsystem
  Compare To Constant2 : simulink/Logic and Bit Operations/Compare To Constant  relop=<  const=0  OutDataTypeStr=boolean
  Constant : Constant  Value=0
  Constant1 : Constant  Value=0
  Constant2 : Constant  Value=0
  Divide1 : Product  Inputs=**
  Logical Operator : Logic  AllPortsSameDT=off  OutDataTypeStr=boolean
  Logical Operator1 : Logic  Operator=OR  AllPortsSameDT=off  OutDataTypeStr=boolean
  MinMax : MinMax  Inputs=2
  MotTRQCAL : Constant
  Motor Torque Available : Subsystem
  NoMotTrqReq : Constant  Value=0
  NoMotTrqReq1 : Constant  Value=0
  SOC Window Estimation : Subsystem
  Shifter : MultiPortSwitch  DataPortOrder=Zero-based contiguous  Inputs=5  zeroidx=on
  Switch1 : Switch  Criteria=u2 > Threshold
  Switch2 : Switch  Criteria=u2 > Threshold  Threshold=1000
  Switch3 : Switch  Criteria=u2 > Threshold
  MotTrq : Outport
  wires:
  [Chg] -> Switch1/2
  MotSpd/1 -> Switch2/2
  Motor Torque Available/1(MotTrqAvl) -> MinMax/2
  APP/1 -> Motor Torque Available/2(APP)
  TransRatio/1 -> Motor Torque Available/1(TransRatio)
  [Chg] -> Compare To Constant2/1
  [MotTrq] -> Switch3/3
  Switch1/1 -> [MotTrq]
  Trq/1 -> Add/1
  Divide1/1 -> [TrqCalc]
  MotTRQCAL/1 -> Divide1/2
  NoMotTrqReq1/1 -> Switch2/3
  Switch2/1 -> Divide1/1
  CS_Switch/1(Out1) -> Logical Operator1/2
  CS_On/1 -> CS_Switch/3(CS_On)
  Faked_SoC/1 -> CS_Switch/2(Faked_SoC_limit)
  SOC Window Estimation/1(Out1) -> Logical Operator1/1
  Logical Operator1/1 -> Logical Operator/2
  Switch3/1 -> Switch2/1
  [Chg] -> Switch3/1
  Logical Operator/1 -> Switch3/2
  Compare To Constant2/1 -> Logical Operator/1
  NoMotTrqReq/1 -> Switch1/3
  MinMax/1 -> Switch1/1
  Add/1 -> MinMax/1, [Chg]
  SoC/1 -> CS_Switch/1(SOC), SOC Window Estimation/1(SOC)
  DrvIntdAxleTrq/1 -> Add/2
  Shifter/1 -> MotTrq/1
  Constant2/1 -> Shifter/5  "N"
  Constant1/1 -> Shifter/3  "P"
  Constant/1 -> Shifter/2  "Between Ranges"
  [TrqCalc] -> Shifter/6  "D"
  [TrqCalc] -> Shifter/4  "R"
  ShftLvrPos/1 -> Shifter/1

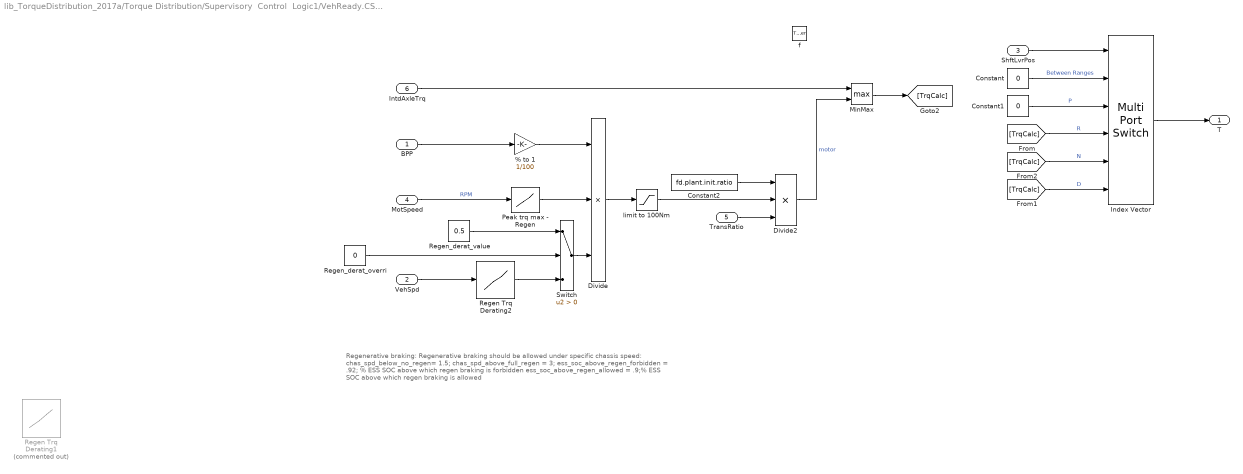
== system lib_TorqueDistribution_2017a/Torque Distribution/Supervisory  Control  Logic1/VehReady.CS_Mode.Motor_Assist.Brake_mode.MotTrqCalc1 ==
  note: Regenerative braking:
      | Regenerative braking should be allowed under specific chassis speed:
      | chas_spd_below_no_regen= 1.5;
      | chas_spd_above_full_regen = 3;
      | ess_soc_above_regen_forbidden = .92;  % ESS SOC above which regen braking is forbidden
      | ess_soc_above_regen_allowed = .9;% ESS SOC above which regen braking is allowed
  BPP : Inport
  VehSpd : Inport  Port=2
  ShftLvrPos : Inport  Port=3
  MotSpeed : Inport  Port=4
  TransRatio : Inport  Port=5
  IntdAxleTrq : Inport  Port=6
  f : TriggerPort  TriggerType=function-call  VariantControl=Variant
      settings: CopyFcn=Stateflow.SLINSF.SimulinkMan.removeBlockPreDeleteFcn  PreDeleteFcn=Stateflow.SLINSF.SimulinkMan.unsafePredeleteFcn
  "% to 1 " : Gain  Gain=1/100
  Constant : Constant  Value=0
  Constant1 : Constant  Value=0
  Constant2 : Constant  Value=fd.plant.init.ratio
  Divide : Product  Inputs=***
  Divide2 : Product  Inputs=***
  Index Vector : MultiPortSwitch  DataPortOrder=Zero-based contiguous  Inputs=5  zeroidx=on
  MinMax : MinMax  Function=max  Inputs=2
  Peak trq max - Regen : Lookup  InputValues=mot.plant.init.regen.trq_max.idx1_spd  Table=mot.plant.init.regen.trq_max.map  LookUpMeth=Interpolation-Use End Values  SaturateOnIntegerOverflow=on
  Regen Trq Derating1 : Lookup_n-D  Commented=on  NumberOfTableDimensions=1  BreakpointsForDimension1=[0 10 20 30 40]  Table=[0 0.025 0.05 0.1 1]  ExtrapMethod=Clip  UseLastTableValue=on  InternalRulePriority=Speed  RndMeth=Simplest  InputSameDT=on
  Regen Trq Derating2 : Lookup_n-D  NumberOfTableDimensions=1  BreakpointsForDimension1=[0 10 11 200]  Table=[0 0.5 1 1]  ExtrapMethod=Clip  UseLastTableValue=on  InternalRulePriority=Speed  RndMeth=Simplest  InputSameDT=on
  Regen_derat_overri : Constant  Value=0
  Regen_derat_value : Constant  Value=0.5
  Switch : Switch  Criteria=u2 > Threshold
  limit to 100Nm : Saturate  UpperLimit=0  LowerLimit=-100
  T : Outport
  wires:
  MinMax/1 -> [TrqCalc]
  IntdAxleTrq/1 -> MinMax/1
  Regen_derat_value/1 -> Switch/1
  Switch/1 -> Divide/3
  Regen_derat_overri/1 -> Switch/2
  Regen Trq Derating2/1 -> Switch/3
  Divide2/1 -> MinMax/2  "motor"
  TransRatio/1 -> Divide2/3
  limit to 100Nm/1 -> Divide2/2
  Constant2/1 -> Divide2/1
  Peak trq max - Regen/1 -> Divide/2
  MotSpeed/1 -> Peak trq max - Regen/1  "RPM"
  [TrqCalc] -> Index Vector/5  "N"
  Constant1/1 -> Index Vector/3  "P"
  Constant/1 -> Index Vector/2  "Between Ranges"
  Index Vector/1 -> T/1
  [TrqCalc] -> Index Vector/6  "D"
  [TrqCalc] -> Index Vector/4  "R"
  ShftLvrPos/1 -> Index Vector/1
  VehSpd/1 -> Regen Trq Derating2/1
  Divide/1 -> limit to 100Nm/1
  "% to 1 "/1 -> Divide/1
  BPP/1 -> "% to 1 "/1

== system lib_TorqueDistribution_2017a/Torque Distribution/Supervisory  Control  Logic1/VehReady.CS_Mode.Motor_Assist.Brake_mode.MotTrqCalc2 ==
  note: Regenerative braking:
      | Regenerative braking should be allowed under specific chassis speed:
      | chas_spd_below_no_regen= 1.5;
      | chas_spd_above_full_regen = 3;
      | ess_soc_above_regen_forbidden = .92;  % ESS SOC above which regen braking is forbidden
      | ess_soc_above_regen_allowed = .9;% ESS SOC above which regen braking is allowed
  ShftLvrPos : Inport
  TransRatio : Inport  Port=2
  f : TriggerPort  TriggerType=function-call  VariantControl=Variant
      settings: CopyFcn=Stateflow.SLINSF.SimulinkMan.removeBlockPreDeleteFcn  PreDeleteFcn=Stateflow.SLINSF.SimulinkMan.unsafePredeleteFcn
  Constant : Constant  Value=0
  Constant1 : Constant  Value=0
  Constant2 : Constant  Value=fd.plant.init.ratio
  Divide2 : Product  Inputs=***
  Idle_torque_Regen : Constant  Value=0
  Index Vector : MultiPortSwitch  DataPortOrder=Zero-based contiguous  Inputs=5  zeroidx=on
  T : Outport
  wires:
  Idle_torque_Regen/1 -> Divide2/2
  Divide2/1 -> [TrqCalc]  "motor"
  TransRatio/1 -> Divide2/3
  Constant2/1 -> Divide2/1
  [TrqCalc] -> Index Vector/5  "N"
  Constant1/1 -> Index Vector/3  "P"
  Constant/1 -> Index Vector/2  "Between Ranges"
  Index Vector/1 -> T/1
  [TrqCalc] -> Index Vector/6  "D"
  [TrqCalc] -> Index Vector/4  "R"
  ShftLvrPos/1 -> Index Vector/1

== system lib_TorqueDistribution_2017a/Torque Distribution/Supervisory  Control  Logic1/VehReady.CS_Mode.Motor_Assist.Drive_mode.MotTrqCalc2 ==
  APP : Inport
  DrvIntdAxleTrq : Inport  Port=2
  TransRatio : Inport  Port=3
  ShftLvrPos : Inport  Port=4
  f : TriggerPort  TriggerType=function-call  VariantControl=Variant
      settings: CopyFcn=Stateflow.SLINSF.SimulinkMan.removeBlockPreDeleteFcn  PreDeleteFcn=Stateflow.SLINSF.SimulinkMan.unsafePredeleteFcn
  Constant : Constant  Value=0
  Constant1 : Constant  Value=0
  Constant2 : Constant  Value=0
  Constant4 : Constant  Value=fd.plant.init.ratio
  Divide2 : Product  Inputs=***
  Index Vector : MultiPortSwitch  DataPortOrder=Zero-based contiguous  Inputs=5  zeroidx=on
  MinMax : MinMax  Inputs=2
  No Torque : Constant  Value=0
  Switch : Switch  Criteria=u2 > Threshold
  drvAPP2CmbTrq : Lookup_n-D  NumberOfTableDimensions=1  BreakpointsForDimension1=[0:1:100]  Table="[5.56903344175488\t20.4825939726242\t30.8750936087224\t37.8858960156155\t42.4930407106164\t45.5262617447488\t47.6795267594729\t49.5230964181710\t51.5151042123953\t54.0126566428754\t57.2824537752881\t61.5109301707869\t66.8139161912932\t73.2458196795481\t80.8083280139256\t89.4586305380063\t99.1171613649123\t109.674862556403\t120.999967676731\t132.944305721263\t145.349125419852\t158.050439914986\t170.883891814679\t183.689138620140\t196.313758528191\t208.616676608453\t220.471111355289\t231.767041614511\t242.413193884843\t252.338549994152\t261.493375150436\t269.849766367567\t277.401721265812\t284.164727247094\t290.174871045030\t295.487468649722\t300.175215607313\t304.325857694294\t308.039381966595\t311.424728183407\t314.596020605783\t317.668320170009\t320.752897035709\t323.952023508727\t327.353287338782\t331.023425391852\t335.001677697353\t339.292661870046\t343.858767906758\t348.612073357775\t353.405778873103\t358.025164123398\t362.178064095715\t365.484865763984\t367.468025134290\t367.541104664833\t364.997331060762\t364.997331060762\t364.997331060762\t364.997331060762\t364.997331060762\t364.997331060762\t364.997331060762\t364.997331060762\t364.997331060762\t364.997331060762\t364.997331060762\t364.997331060762\t364.997331060762\t364.997331060762\t364.997331060762\t364.997331060762\t364.997331060762\t364.997331060762\t364.997331060762\t364.997331060762\t364.997331060762\t364.997331060762\t364.997331060762\t364.997331060762\t364.997331060762\t364.997331060762\t364.997331060762\t364.997331060762\t364.997331060762\t364.997331060762\t364.997331060762\t364.997331060762\t364.997331060762\t364.997331060762\t364.997331060762\t364.997331060762\t364.997331060762\t364.997331060762\t364.997331060762\t364.997331060762\t364.997331060762\t364.997331060762\t364.997331060762\t364.997331060762\t364.997331060762]"  ExtrapMethod=Clip  UseLastTableValue=on  InternalRulePriority=Speed  RndMeth=Simplest  InputSameDT=on
  MotTrq : Outport
  wires:
  APP/1 -> drvAPP2CmbTrq/1, Switch/2
  Switch/1 -> MinMax/2  "MotAvlTrq"
  Divide2/1 -> Switch/1
  No Torque/1 -> Switch/3
  DrvIntdAxleTrq/1 -> MinMax/1
  TransRatio/1 -> Divide2/1
  MinMax/1 -> [TrqCalc]
  drvAPP2CmbTrq/1 -> Divide2/3
  Constant4/1 -> Divide2/2
  Index Vector/1 -> MotTrq/1
  Constant2/1 -> Index Vector/5  "N"
  Constant1/1 -> Index Vector/3  "P"
  Constant/1 -> Index Vector/2  "Between Ranges"
  [TrqCalc] -> Index Vector/6  "D"
  [TrqCalc] -> Index Vector/4  "R"
  ShftLvrPos/1 -> Index Vector/1
